simulink model "Esquema_PSK"  (R2020b)
settings: Solver=VariableStepAuto  StartTime=0.0  StopTime=Timesim  RelTol=1e-3
values from neighbouring files (symbols this model uses):
  Amplitud = 1    [Parametros_PSK.m]
  Ancho_banda_minimo = Rb    (= 50000)    [Parametros_PSK.m]
  Att_pot_Canal = 10^(Att_dB / 10)    [Parametros_PSK.m]
  Att_Volt_Canal = 10^(Att_dB / 20)    [Parametros_PSK.m]
  b = 0.6    [Parametros_PSK.m]
  C = 1e-6    (= 1e-06)    [Parametros_PSK.m]
  Frec_port = 1000000    [Parametros_PSK.m]
  Kv = 2 * pi * 1E6    (= 6283185.30718)    [Parametros_PSK.m]
  Pot_Ruido = eta * Ancho_banda_minimo    [Parametros_PSK.m]
  R1 = Kp * Kv / (wn^2 * C)    (= 2.48224604728)    [Parametros_PSK.m]
  R2 = 2 * zeta / (wn * C)    (= 1.42222222222)    [Parametros_PSK.m]
  Rb = 50000    [Parametros_PSK.m]
  Retraso_Canal = Long_Canal / C_canal    (= 0.0001)    [Parametros_PSK.m]
  Retraso_total = Retraso_Canal + Retraso_filtro    (= 0.000115)    [Parametros_PSK.m]
  Umbral = 0    [Parametros_PSK.m]
libraries: dspsigops x6, simulink_extras x4, dsparch4 x4, commsynccomp2 x2, powerlib_extras x2, dspsnks4 x2, simulink x1
settings Model: Creator=PedroPablo  LastModifiedBy=DPK

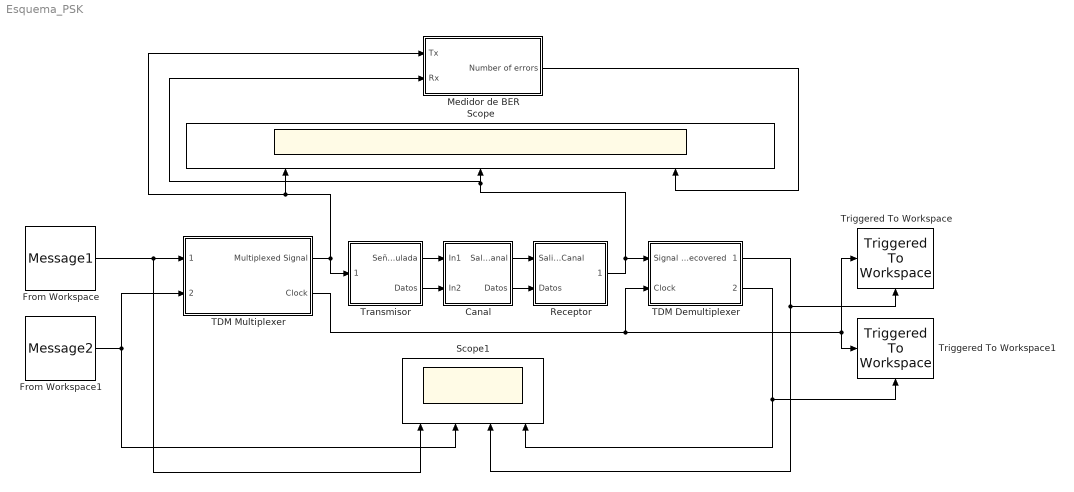
== system Esquema_PSK ==
  Canal : Subsystem
  From Workspace : FromWorkspace  VariableName=Message1  OutDataTypeStr=double  SampleTime=2/Rb  Interpolate=off  OutputAfterFinalValue=Setting to zero
  From Workspace1 : FromWorkspace  VariableName=Message2  OutDataTypeStr=double  SampleTime=2/Rb  Interpolate=off  OutputAfterFinalValue=Setting to zero
  Medidor de BER : Subsystem
  Receptor : Subsystem
  Scope : Scope  NumInputPorts=3
  Scope1 : Scope  NumInputPorts=4
  TDM Demultiplexer : Subsystem
  TDM Multiplexer : Subsystem
  Transmisor : Subsystem
  Triggered To Workspace : dspsnks4/Triggered To Workspace  TriggerType=Rising edge  VariableName=Salida1  Buffer=1000  Save2DMode=2-D array (concatenate along first dimension)
      settings: SourceProductBaseCode=DS  FixptAsFi=off
  Triggered To Workspace1 : dspsnks4/Triggered To Workspace  TriggerType=Rising edge  VariableName=Salida2  Buffer=1000  Save2DMode=2-D array (concatenate along first dimension)
      settings: SourceProductBaseCode=DS  FixptAsFi=off
  wires:
  Transmisor/1(Señal modulada) -> Canal/1(In1)
  Transmisor/2(Datos) -> Canal/2(In2)
  Canal/1(Salida Canal) -> Receptor/1(Salida Canal)
  Canal/2(Datos) -> Receptor/2(Datos)
  From Workspace1/1 -> Scope1/2, TDM Multiplexer/2(2)
  From Workspace/1 -> Scope1/1, TDM Multiplexer/1(1)
  TDM Demultiplexer/1(" 1") -> Scope1/3, Triggered To Workspace/1
  TDM Demultiplexer/2(" 2") -> Scope1/4, Triggered To Workspace1/1
  TDM Multiplexer/2(Clock) -> Triggered To Workspace/Trigger, Triggered To Workspace1/Trigger, TDM Demultiplexer/2(Clock)
  TDM Multiplexer/1(Multiplexed Signal) -> Transmisor/1(1), Medidor de BER/1(Tx), Scope/1
  Receptor/1(1) -> TDM Demultiplexer/1(Signal Recovered), Medidor de BER/2(Rx), Scope/2
  Medidor de BER/1(Number of errors) -> Scope/3

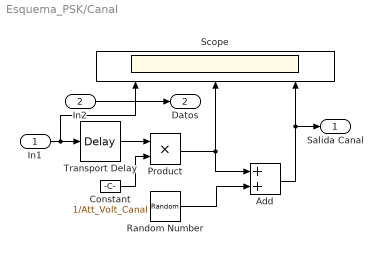
== system Esquema_PSK/Canal ==
  In1 : Inport
  In2 : Inport  Port=2
  Add : Sum
  Constant : Constant  Value=1/Att_Volt_Canal
  Product : Product
  Random Number : RandomNumber  Variance=Pot_Ruido  SampleTime=1/(1000*Rb)
  Scope : Scope  NumInputPorts=3
  Transport Delay : TransportDelay  DelayTime=Retraso_Canal
  Salida Canal : Outport
  Datos : Outport  Port=2
  wires:
  In2/1 -> Datos/1
  Product/1 -> Add/1, Scope/2
  Add/1 -> Scope/3, Salida Canal/1
  Constant/1 -> Product/2
  In1/1 -> Scope/1, Transport Delay/1
  Random Number/1 -> Add/2
  Transport Delay/1 -> Product/1

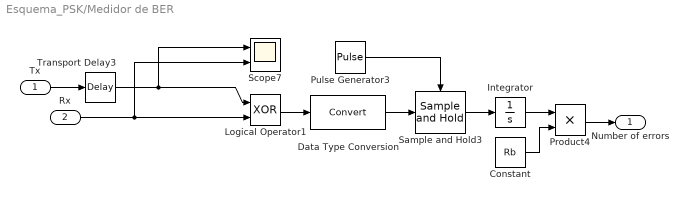
== system Esquema_PSK/Medidor de BER ==
  Tx : Inport
  Rx : Inport  Port=2
  Constant : Constant  Value=Rb
  Data Type Conversion : DataTypeConversion
  Integrator : Integrator
  Logical Operator1 : Logic  Operator=XOR  AllPortsSameDT=off  OutDataTypeStr=boolean
  Product4 : Product
  Pulse Generator3 : DiscretePulseGenerator  PulseType=Time based  Period=1/Rb  PhaseDelay=0.1*(1/Rb)
  Sample and Hold3 : dspsigops/Sample and Hold  trig=Falling edge  initCond=0  latchinput=off
  Scope7 : Scope  NumInputPorts=2
  Transport Delay3 : TransportDelay  DelayTime=133.877e-6
  Number of errors : Outport
  wires:
  Transport Delay3/1 -> Logical Operator1/1, Scope7/1
  Integrator/1 -> Product4/1
  Pulse Generator3/1 -> Sample and Hold3/Trigger
  Logical Operator1/1 -> Data Type Conversion/1
  Tx/1 -> Transport Delay3/1
  Sample and Hold3/1 -> Integrator/1
  Constant/1 -> Product4/2
  Data Type Conversion/1 -> Sample and Hold3/1
  Rx/1 -> Logical Operator1/2, Scope7/2
  Product4/1 -> Number of errors/1

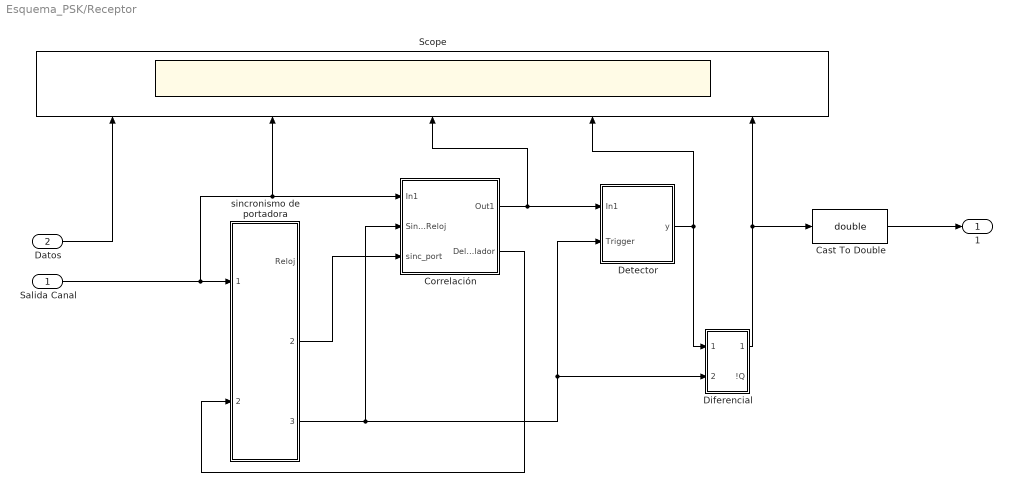
== system Esquema_PSK/Receptor ==
  Salida Canal : Inport
  Datos : Inport  Port=2
  Cast To Double : DataTypeConversion  OutDataTypeStr=double
  Correlación : Subsystem
  Detector : Subsystem
  Diferencial : Subsystem
  Scope : Scope  NumInputPorts=5
  sincronismo de portadora : Subsystem
  1 : Outport
  wires:
  Datos/1 -> Scope/1
  Correlación/1(Out1) -> Detector/1(In1), Scope/3
  Salida Canal/1 -> sincronismo de portadora/1(Salida Canal), Correlación/1(In1), Scope/2
  Detector/1(y) -> Diferencial/1(Datos), Scope/4
  sincronismo de portadora/2(Sinc_port) -> Correlación/3(sinc_port)
  Correlación/2(Del correlador) -> sincronismo de portadora/2(Del correlador)
  sincronismo de portadora/3(Sinc_Reloj) -> Correlación/2(Sinc_Reloj), Diferencial/2(Reloj), Detector/2(Trigger)
  Diferencial/1(Out1) -> Scope/5, Cast To Double/1
  Cast To Double/1 -> 1/1

== system Esquema_PSK/TDM Demultiplexer ==
  Signal Recovered : Inport
  Clock : Inport  Port=2
  Sample and Hold3 : dspsigops/Sample and Hold  trig=Falling edge  initCond=0  latchinput=off
  Sample and Hold4 : dspsigops/Sample and Hold  trig=Rising edge  initCond=0  latchinput=off
  " 1" : Outport
  " 2" : Outport  Port=2
  wires:
  Sample and Hold3/1 -> " 1"/1
  Signal Recovered/1 -> Sample and Hold4/1, Sample and Hold3/1
  Sample and Hold4/1 -> " 2"/1
  Clock/1 -> Sample and Hold4/Trigger, Sample and Hold3/Trigger

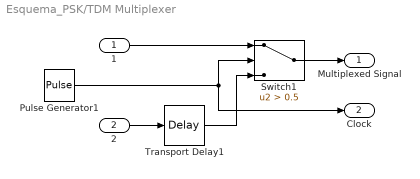
== system Esquema_PSK/TDM Multiplexer ==
  1 : Inport
  2 : Inport  Port=2
  Pulse Generator1 : DiscretePulseGenerator  PulseType=Time based  Period=2/Rb  PulseWidth=50
  Switch1 : Switch  Criteria=u2 > Threshold  Threshold=0.5
  Transport Delay1 : TransportDelay  DelayTime=2/Rb
  Multiplexed Signal : Outport
  Clock : Outport  Port=2
  wires:
  Switch1/1 -> Multiplexed Signal/1
  Transport Delay1/1 -> Switch1/3
  Pulse Generator1/1 -> Clock/1, Switch1/2
  2/1 -> Transport Delay1/1
  1/1 -> Switch1/1

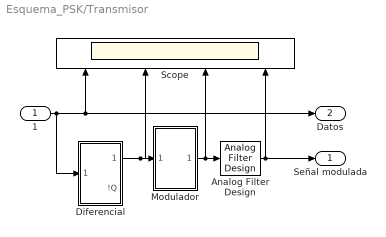
== system Esquema_PSK/Transmisor ==
  1 : Inport
  Analog Filter Design : dsparch4/Analog Filter Design  method=Butterworth  filttype=Bandpass  N=8  Wlo=2*pi*(Frec_port - Ancho_banda_minimo)  Whi=2*pi*(Frec_port + Ancho_banda_minimo)  Rp=2  Rs=40
  Diferencial : Subsystem
  Modulador : Subsystem
  Scope : Scope  NumInputPorts=4
  Señal modulada : Outport
  Datos : Outport  Port=2
  wires:
  1/1 -> Diferencial/1(In1), Datos/1, Scope/1
  Analog Filter Design/1 -> Señal modulada/1, Scope/4
  Modulador/1(Out1) -> Scope/3, Analog Filter Design/1
  Diferencial/1(Out1) -> Scope/2, Modulador/1(In1)

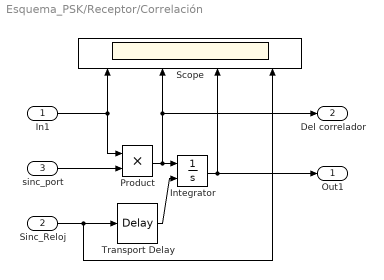
== system Esquema_PSK/Receptor/Correlación ==
  In1 : Inport
  Sinc_Reloj : Inport  Port=2
  sinc_port : Inport  Port=3
  Integrator : Integrator  ExternalReset=rising
  Product : Product
  Scope : Scope  NumInputPorts=4
  Transport Delay : TransportDelay  DelayTime=1e-9
  Out1 : Outport
  Del correlador : Outport  Port=2
  wires:
  Transport Delay/1 -> Integrator/2
  In1/1 -> Product/1, Scope/1
  Integrator/1 -> Out1/1, Scope/3
  Product/1 -> Integrator/1, Del correlador/1, Scope/2
  Sinc_Reloj/1 -> Scope/4, Transport Delay/1
  sinc_port/1 -> Product/2

== system Esquema_PSK/Receptor/Detector ==
  In1 : Inport
  Trigger : Inport  Port=2
  Compare To Constant : simulink/Logic and Bit Operations/Compare To Constant  relop=>=  const=Umbral  OutDataTypeStr=boolean
  Sample and Hold : dspsigops/Sample and Hold  trig=Rising edge  initCond=0  latchinput=off
  Scope : Scope  NumInputPorts=4
  y : Outport
  wires:
  In1/1 -> Sample and Hold/1, Scope/1
  Compare To Constant/1 -> Scope/4, y/1
  Trigger/1 -> Scope/2, Sample and Hold/Trigger
  Sample and Hold/1 -> Scope/3, Compare To Constant/1

== system Esquema_PSK/Receptor/Diferencial ==
  Datos : Inport
  Reloj : Inport  Port=2
  Constant : Constant
  D Flip-Flop : simulink_extras/Flip Flops/D Flip-Flop
  Logical Operator : Logic  Operator=NXOR  AllPortsSameDT=off  OutDataTypeStr=boolean
  Out1 : Outport
  !Q : Outport  Port=2
  wires:
  Reloj/1 -> D Flip-Flop/2
  Logical Operator/1 -> Out1/1
  Constant/1 -> D Flip-Flop/3
  D Flip-Flop/1 -> Logical Operator/1
  Datos/1 -> D Flip-Flop/1, Logical Operator/2
  D Flip-Flop/2 -> !Q/1

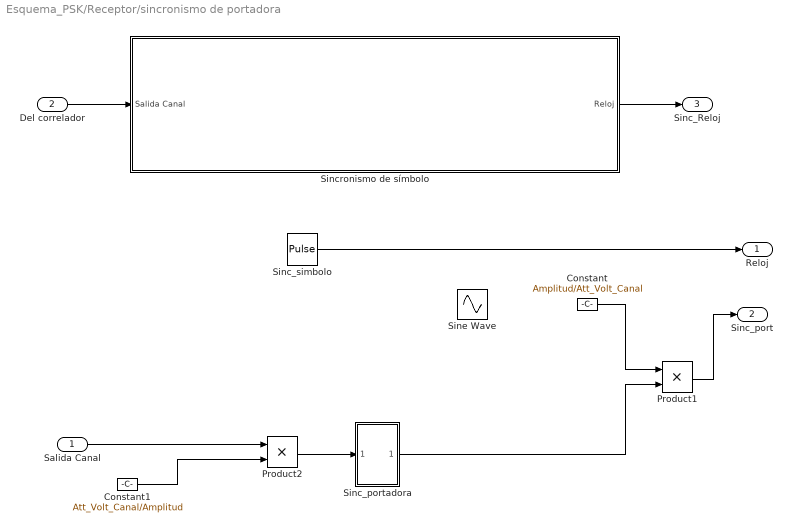
== system Esquema_PSK/Receptor/sincronismo de portadora ==
  Salida Canal : Inport
  Del correlador : Inport  Port=2
  Constant : Constant  Value=Amplitud/Att_Volt_Canal
  Constant1 : Constant  Value=Att_Volt_Canal/Amplitud
  Product1 : Product
  Product2 : Product
  Sinc_portadora : Subsystem
  Sinc_simbolo : DiscretePulseGenerator  PulseType=Time based  Amplitude=Amplitud  Period=1/Rb  PulseWidth=50  PhaseDelay=Retraso_total
  Sincronismo de símbolo : Subsystem
  Sine Wave : Sin  Amplitude=Amplitud/Att_Volt_Canal  Frequency=2*pi*Frec_port  SampleTime=0
  Reloj : Outport
  Sinc_port : Outport  Port=2
  Sinc_Reloj : Outport  Port=3
  wires:
  Constant/1 -> Product1/1
  Product1/1 -> Sinc_port/1
  Sinc_simbolo/1 -> Reloj/1
  Salida Canal/1 -> Product2/1
  Sinc_portadora/1(Out1) -> Product1/2
  Constant1/1 -> Product2/2
  Product2/1 -> Sinc_portadora/1(In1)
  Sincronismo de símbolo/1(Reloj) -> Sinc_Reloj/1
  Del correlador/1 -> Sincronismo de símbolo/1(Salida Canal)

== system Esquema_PSK/Transmisor/Diferencial ==
  In1 : Inport
  Clock : simulink_extras/Flip Flops/Clock  period=Tb
  Constant : Constant
  D Flip-Flop : simulink_extras/Flip Flops/D Flip-Flop
  Logical Operator : Logic  Operator=NXOR  AllPortsSameDT=off  OutDataTypeStr=boolean
  Out1 : Outport
  !Q : Outport  Port=2
  wires:
  Clock/1 -> D Flip-Flop/2
  Logical Operator/1 -> Out1/1, D Flip-Flop/1
  Constant/1 -> D Flip-Flop/3
  D Flip-Flop/1 -> Logical Operator/1
  In1/1 -> Logical Operator/2
  D Flip-Flop/2 -> !Q/1

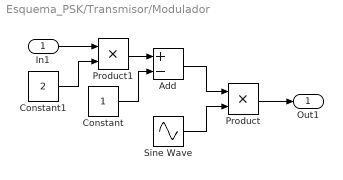
== system Esquema_PSK/Transmisor/Modulador ==
  In1 : Inport
  Add : Sum  Inputs=+-
  Constant : Constant
  Constant1 : Constant  Value=2
  Product : Product
  Product1 : Product
  Sine Wave : Sin  Amplitude=Amplitud  Frequency=2*pi*(Frec_port)  SampleTime=0
  Out1 : Outport
  wires:
  Product/1 -> Out1/1
  Sine Wave/1 -> Product/2
  In1/1 -> Product1/1
  Constant1/1 -> Product1/2
  Product1/1 -> Add/1
  Constant/1 -> Add/2
  Add/1 -> Product/1

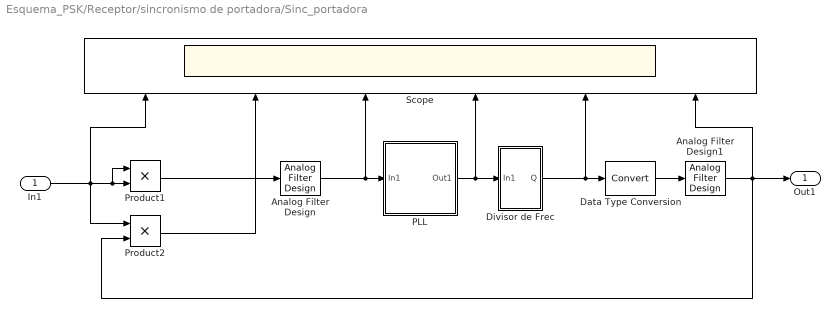
== system Esquema_PSK/Receptor/sincronismo de portadora/Sinc_portadora ==
  In1 : Inport
  Analog Filter Design : dsparch4/Analog Filter Design  method=Butterworth  filttype=Bandpass  N=2  Wlo=2*pi*(2*Frec_port - Ancho_banda_minimo/10)  Whi=2*pi*(2*Frec_port + Ancho_banda_minimo/10)  Rp=2  Rs=40
  Analog Filter Design1 : dsparch4/Analog Filter Design  method=Butterworth  filttype=Bandpass  N=8  Wlo=2*pi*(Frec_port - Ancho_banda_minimo)  Whi=2*pi*(Frec_port + Ancho_banda_minimo)  Rp=2  Rs=40
  Data Type Conversion : DataTypeConversion
  Divisor de Frec : Subsystem
  PLL : Subsystem
  Product1 : Product
  Product2 : Product
  Scope : Scope  NumInputPorts=6
  Out1 : Outport
  wires:
  In1/1 -> Product2/1, Scope/1, Product1/2, Product1/1
  Product1/1 -> Analog Filter Design/1
  Analog Filter Design/1 -> PLL/1(In1), Scope/3
  PLL/1(Out1) -> Divisor de Frec/1(In1), Scope/4
  Divisor de Frec/1(Q) -> Data Type Conversion/1, Scope/5
  Analog Filter Design1/1 -> Out1/1, Product2/2, Scope/6
  Data Type Conversion/1 -> Analog Filter Design1/1
  Product2/1 -> Scope/2

== system Esquema_PSK/Receptor/sincronismo de portadora/Sincronismo de símbolo ==
  Salida Canal : Inport
  AGC1 : Subsystem
  Analog Filter Design : dsparch4/Analog Filter Design  method=Butterworth  filttype=Bandpass  N=2  Wlo=2*pi*(Rb/2- Ancho_banda_minimo/100)  Whi=2*pi*(Rb/2+ Ancho_banda_minimo/100)  Rp=2  Rs=40
  Early_Late : Subsystem
  Scope : Scope  NumInputPorts=3
  Sign : Signum
  Reloj : Outport
  wires:
  Salida Canal/1 -> AGC1/1(In1)
  Early_Late/1(Reloj) -> Reloj/1
  Sign/1 -> Scope/3, Early_Late/1(In1)
  AGC1/1(Out1) -> Scope/1, Analog Filter Design/1
  Analog Filter Design/1 -> Sign/1, Scope/2

== system Esquema_PSK/Receptor/sincronismo de portadora/Sinc_portadora/Divisor de Frec ==
  In1 : Inport
  Constant2 : Constant
  D Flip-Flop : simulink_extras/Flip Flops/D Flip-Flop
  Sign : Signum
  Q : Outport
  wires:
  D Flip-Flop/1 -> Q/1
  Constant2/1 -> D Flip-Flop/3
  D Flip-Flop/2 -> D Flip-Flop/1
  In1/1 -> Sign/1
  Sign/1 -> D Flip-Flop/2

== system Esquema_PSK/Receptor/sincronismo de portadora/Sinc_portadora/PLL ==
  note: 0.125/Frec_port o 4.475e-9
  In1 : Inport
  Continuous-Time VCO : commsynccomp2/Continuous-Time VCO  Ac=Amplitud/Att_Volt_Canal  Fc=2*Frec_port  Kc=Kv/(2*pi)  Ph=pi/2
      settings: SourceProductBaseCode=CM
  Loop Filter : Subsystem
  Transport Delay : TransportDelay  DelayTime=0.5/Frec_port
  phase Detector : Product
  Out1 : Outport
  wires:
  phase Detector/1 -> Loop Filter/1(In1)
  Continuous-Time VCO/1 -> phase Detector/2, Transport Delay/1
  Transport Delay/1 -> Out1/1
  In1/1 -> phase Detector/1
  Loop Filter/1(Out1) -> Continuous-Time VCO/1

== system Esquema_PSK/Receptor/sincronismo de portadora/Sincronismo de símbolo/AGC1 ==
  In1 : Inport
  Constant1 : Constant  Value=Att_pot_Canal/(Amplitud^2)
  Product2 : Product
  Out1 : Outport
  wires:
  In1/1 -> Product2/2
  Product2/1 -> Out1/1
  Constant1/1 -> Product2/1

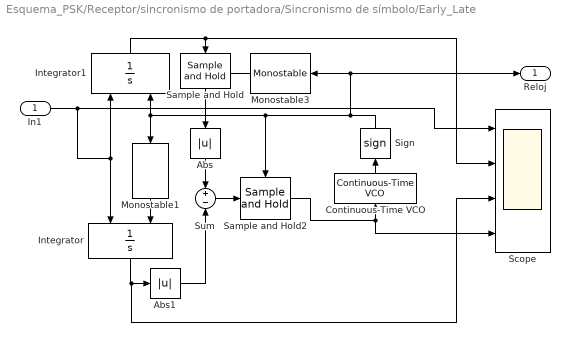
== system Esquema_PSK/Receptor/sincronismo de portadora/Sincronismo de símbolo/Early_Late ==
  In1 : Inport
  Abs : Abs
  Abs1 : Abs
  Continuous-Time VCO : commsynccomp2/Continuous-Time VCO  Ac=1  Fc=Rb  Kc=kv2  Ph=0
      settings: SourceProductBaseCode=CM
  Integrator : Integrator  ExternalReset=falling  UpperSaturationLimit=0.7e-4  LowerSaturationLimit=-0.7e-4
  Integrator1 : Integrator  ExternalReset=rising  UpperSaturationLimit=0.7e-4  LowerSaturationLimit=-0.7e-4
  Monostable1 : powerlib_extras/Control  Blocks/Monostable  EdgeDetect=Rising  t_mono=(1-b)/Rb  ic=0
      settings: SourceProductBaseCode=PS
  Monostable3 : powerlib_extras/Control  Blocks/Monostable  EdgeDetect=Rising  t_mono=b/Rb  ic=0
      settings: SourceProductBaseCode=PS
  Sample and Hold : dspsigops/Sample and Hold  trig=Falling edge  initCond=0  latchinput=off
  Sample and Hold2 : dspsigops/Sample and Hold  trig=Rising edge  initCond=0  latchinput=off
  Scope : Scope  NumInputPorts=4
  Sign : Signum
  Sum : Sum  Inputs=+-
  Reloj : Outport
  wires:
  Monostable1/1 -> Integrator/2
  Monostable3/1 -> Sample and Hold/Trigger
  Integrator/1 -> Scope/3, Abs1/1
  Sample and Hold/1 -> Abs/1
  Abs1/1 -> Sum/2
  Integrator1/1 -> Scope/2, Sample and Hold/1
  Sum/1 -> Sample and Hold2/1
  Abs/1 -> Sum/1
  Sign/1 -> Integrator1/2, Monostable1/1, Sample and Hold2/Trigger, Reloj/1, Monostable3/1
  Continuous-Time VCO/1 -> Sign/1
  In1/1 -> Scope/1, Integrator/1, Integrator1/1
  Sample and Hold2/1 -> Continuous-Time VCO/1, Scope/4

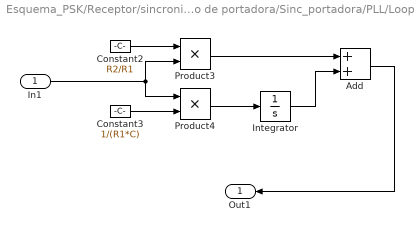
== system Esquema_PSK/Receptor/sincronismo de portadora/Sinc_portadora/PLL/Loop Filter ==
  In1 : Inport
  Add : Sum
  Constant2 : Constant  Value=R2/R1
  Constant3 : Constant  Value=1/(R1*C)
  Integrator : Integrator
  Product3 : Product
  Product4 : Product
  Out1 : Outport
  wires:
  Add/1 -> Out1/1
  Constant3/1 -> Product4/2
  Integrator/1 -> Add/2
  Product4/1 -> Integrator/1
  In1/1 -> Product3/2, Product4/1
  Product3/1 -> Add/1
  Constant2/1 -> Product3/1
